simulink model "AirplaneSimModel_AutomaticTrajectory"  (R2018b)
settings: Solver=ode4  StartTime=0.0  StopTime=30  FixedStep=0.001  RelTol=1e-3
undefined symbols (not defined in the file): aileron_left, aileron_right, airplane, alt_ground, atmosphere, B_aileron_p_14ms, B_elevator_q_14ms, B_rudder_r_14ms, elevator, envir, g, htp_trim, inital_vel_vec, K_atti, K_lateral, K_vertical, rudder, throttle, traj, wind
libraries: actuators_lib x11, unit_conversions_lib x6, axes_transformation_lib x2, quatAttitudeController_lib x2, conventional_airplane_single_engine_lib x1, atmosphere_lib x1, sensors_lib x1, simulink x1, flightgear_visualization_lib x1
(part 1 of 2)
settings Model: Creator=Fgücker  LastModifiedBy=fabian

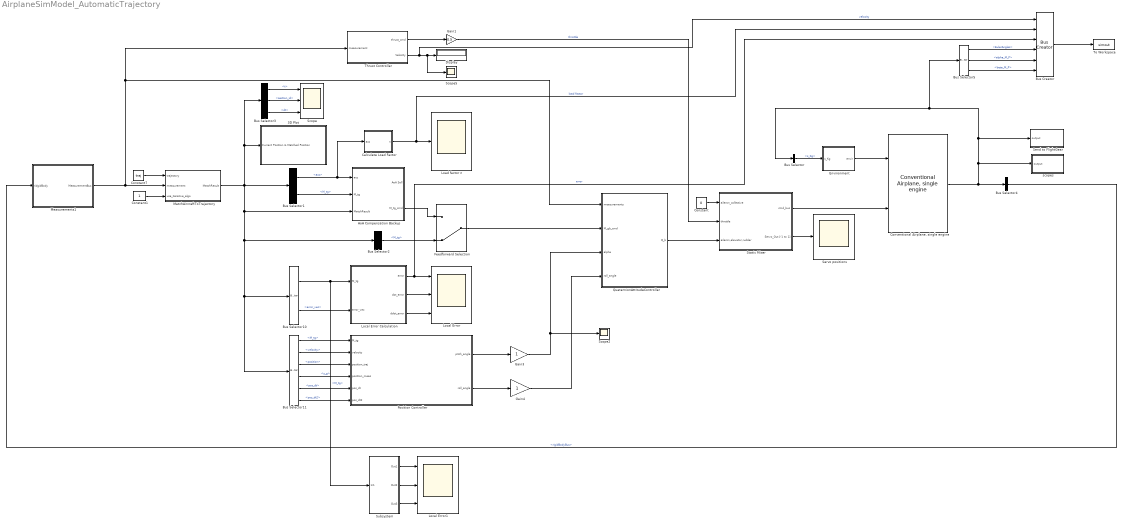
== system AirplaneSimModel_AutomaticTrajectory ==
  3D Plot : Subsystem
  AoA Compensation Backup : Subsystem
  Bus Creator : BusCreator  Inputs=6
  Bus Selector : BusSelector  OutputSignals=rigidBodyBus.s_Kg
  Bus Selector1 : BusSelector  OutputSignals=acc,M_tg
  Bus Selector10 : BusSelector  OutputSignals=M_tg,error_vec
  Bus Selector11 : BusSelector  OutputSignals=M_tg,velocity,position,s_g,pos_dt,pos_dt2
  Bus Selector2 : BusSelector  OutputSignals=M_tg
  Bus Selector3 : BusSelector  OutputSignals=t,section_id,dt
  Bus Selector4 : BusSelector  OutputSignals=rigidBodyBus
  Bus Selector5 : BusSelector  OutputSignals=rigidBodyBus.EulerAngles,aeroBus.aeroMainWing.aeroAxes.alpha_M_P,aeroBus.aeroMainWing.aeroAxes.beta_M_P
  Calculate Load Factor : Subsystem
  Constant : Constant  Value=0
  Constant1 : Constant
  Constant7 : Constant  Value=traj  OutDataTypeStr=Bus: trajectoryBus
  "Conventional Airplane, single engine" : conventional_airplane_single_engine_lib/Conventional Airplane, single engine  airplane=airplane
      settings: SourceProductName=LADAC
  Display : Display
  Environment : Subsystem
  Feedforward Selection : ManualSwitch  CurrentSetting=0
  Gain1 : Gain  Gain=0.5
  Gain3 : Gain
  Gain4 : Gain
  Load factor n : Scope
  Local Error : Scope  NumInputPorts=3
  Local Error Calculation : Subsystem
  Local Error1 : Scope  NumInputPorts=3
  MatchAircraftToTrajectory : Subsystem
  Measurements1 : Subsystem  mask{omega0=80, D=1}
      mask prompts: omega0 "Omega - Filter"; D "Damping D - Filter"
  Position Controller : Subsystem
  QuaternionAttitudeController : Subsystem
  Scope : Scope  NumInputPorts=3
  Scope2 : Scope
  Scope5 : Scope
  Send to FlightGear : Subsystem
  Servo positions : Scope
  Static Mixer : Subsystem
  Subsystem : Subsystem
  Thrust Controller : Subsystem
  To Workspace : ToWorkspace  VariableName=simout  SaveFormat=Timeseries  SampleTime=-1
  scopes : Subsystem
  wires:
  Bus Selector4/1 -> Measurements1/1(ridgidBody)  "<rigidBodyBus>"
  Measurements1/1(MeasurementBus) -> Thrust Controller/1(measurement), QuaternionAttitudeController/1(measurements), MatchAircraftToTrajectory/2(measurement)
  Thrust Controller/1(thrust_cmd) -> Gain1/1
  Thrust Controller/2(Velocity) -> Bus Creator/1, Scope5/1, Display/1  "velocity"
  AoA Compensation Backup/2(M_tg_cmd) -> Feedforward Selection/1
  "Conventional Airplane, single engine"/1 -> Bus Selector4/1, Bus Selector5/1, Bus Selector/1, Send to FlightGear/1(output), scopes/1(output)
  Environment/1(envir) -> "Conventional Airplane, single engine"/1
  Bus Selector/1 -> Environment/1(s_Kg)  "<s_Kg>"
  Feedforward Selection/1 -> QuaternionAttitudeController/2(M_gb_cmd)
  Bus Selector11/2 -> Position Controller/2(velocity)  "<velocity>"
  Bus Selector11/3 -> Position Controller/3(position_traj)  "<position>"
  Local Error Calculation/3(ddot_error) -> Local Error/3
  Local Error Calculation/2(dot_error) -> Local Error/2
  Local Error Calculation/1(error) -> Bus Creator/3, Local Error/1  "error"
  Bus Selector10/2 -> Local Error Calculation/2(error_vec)  "<error_vec>"
  Gain1/1 -> Static Mixer/2(throttle)  "throttle"
  QuaternionAttitudeController/1(Q_b) -> Static Mixer/3(aileron,elevator,rudder)
  Static Mixer/1(cmd_bus) -> "Conventional Airplane, single engine"/2
  Static Mixer/2(Servo_Out [-1 to 1]) -> Servo positions/1
  Constant7/1 -> MatchAircraftToTrajectory/1(trajectory)
  Bus Selector11/1 -> Position Controller/1(M_tg)  "<M_tg>"
  Bus Selector10/1 -> Subsystem/1(In1), Local Error Calculation/1(M_tg)  "<M_tg>"
  Bus Selector11/4 -> Position Controller/4(position_meas)  "<s_g>"
  Calculate Load Factor/1(n) -> Bus Creator/2, Load factor n/1  "load factor"
  Bus Selector1/1 -> AoA Compensation Backup/1(acc), Calculate Load Factor/1(acc)  "<acc>"
  Bus Selector1/2 -> AoA Compensation Backup/2(M_tg)  "<M_tg>"
  Bus Selector2/1 -> Feedforward Selection/2  "<M_tg>"
  Constant/1 -> Static Mixer/1(aileron_collective)
  Bus Selector3/1 -> Scope/1  "<t>"
  Bus Selector3/2 -> Scope/2  "<section_id>"
  Subsystem/1(Out1) -> Local Error1/1
  Subsystem/2(Out2) -> Local Error1/2
  Subsystem/3(Out3) -> Local Error1/3
  Gain3/1 -> Scope2/1, QuaternionAttitudeController/3(alpha)
  Gain4/1 -> QuaternionAttitudeController/4(roll_angle)
  Bus Creator/1 -> To Workspace/1
  Bus Selector5/1 -> Bus Creator/4  "<EulerAngles>"
  Bus Selector5/2 -> Bus Creator/5  "<alpha_M_P>"
  Bus Selector5/3 -> Bus Creator/6  "<beta_M_P>"
  Constant1/1 -> MatchAircraftToTrajectory/3(use_iterative_algo)
  Bus Selector11/5 -> Position Controller/5(pos_dt)  "<pos_dt>"
  Bus Selector11/6 -> Position Controller/6(pos_dt2)  "<pos_dt2>"
  MatchAircraftToTrajectory/1(MatchResult) -> Bus Selector11/1, Bus Selector10/1, Bus Selector2/1, AoA Compensation Backup/3(MatchResult), Bus Selector1/1, Bus Selector3/1, 3D Plot/1(Current Position & Matched Position)
  Position Controller/1(pitch_angle) -> Gain3/1
  Position Controller/2(roll_angle) -> Gain4/1
  Bus Selector3/3 -> Scope/3  "<dt>"

== system AirplaneSimModel_AutomaticTrajectory/3D Plot ==
  Current Position & Matched Position : Inport
  3D Graph : S-Function  LoadFcn=if exist('sfun3d','file'), sfun3d([],[],[],'LoadBlock'); end  FunctionName=sfun3d  Parameters=ax,T,np,cp,gd,ls,mk,mx,hd,tb  SFunctionDeploymentMode=off  EnableBusSupport=off  mask(3D Graph){np=2, ax=[-8 8 -8 8 -8 8]*20, mx=1e4, T=0.040, cp=[-1 -1 1]*35, gd=on, hd=off, tb=off, ls=-, mk=none}
      mask prompts: np "Number of moving points (lines)"; ax "Range: [xmin xmax  ymin ymax zmin zmax]"; mx "Max number of points in each line"; T "Sampling Time"; cp "Camera position (use [0 0 1] for 2D XY view)"; gd "Grid (on|off)"; hd "HeadMarkers (on|off)"; tb "Toolbar (on|off)"; ls "LineStyle"; mk "LineMarker"
      mask help:
      | This block plots the position of several points in the XYZ space. The input contains the coordinates of all the points (x1,y1,z1,x2,y2,z2,...).
      | The number of moving points (lines), the XYZ ranges, sampling time, camera position, and grid (among other things) can be set as mask parameters.
      settings: CopyFcn=if exist('sfun3d','file'), sfun3d([],[],[],'CopyBlock'); end  DeleteFcn=if exist('sfun3d','file'), sfun3d([],[],[],'DeleteBlock'); end  NameChangeFcn=if exist('sfun3d','file'), sfun3d([],[],[],'NameChange'); end
      mask Help:
      | This block plots the position of several points in the XYZ space. The input contains the coordinates of all the points (x1,y1,z1,x2,y2,z2,...).
      | The number of moving points (lines), the XYZ ranges, sampling time, camera position, and grid (among other things) can be set as mask parameters.
      mask TypeOptions ls: - | -- | : | -. | none
      mask TypeOptions mk: none | . | + | o | * | x | square | diamond | v | ^ | > | < | pentagram | hexagram
      mask Display: plot([.05 .95 .95 .05 .05],[.45 .45 .95 .95 .45], 0.5+cos(0:0.1:2*pi)*0.3,0.7+sin(0:0.1:2*pi)*0.2)
  Bus Selector5 : BusSelector  OutputSignals=s_g,position
  Gain19 : Gain  Gain=[1 1 -1]'
  Gain2 : Gain  Gain=[1 1 -1]'
  Mux : Mux  Inputs=2
  wires:
  Bus Selector5/2 -> Gain19/1  "<position>"
  Gain19/1 -> Mux/2
  Current Position & Matched Position/1 -> Bus Selector5/1
  Bus Selector5/1 -> Gain2/1  "<s_g>"
  Mux/1 -> 3D Graph/1
  Gain2/1 -> Mux/1

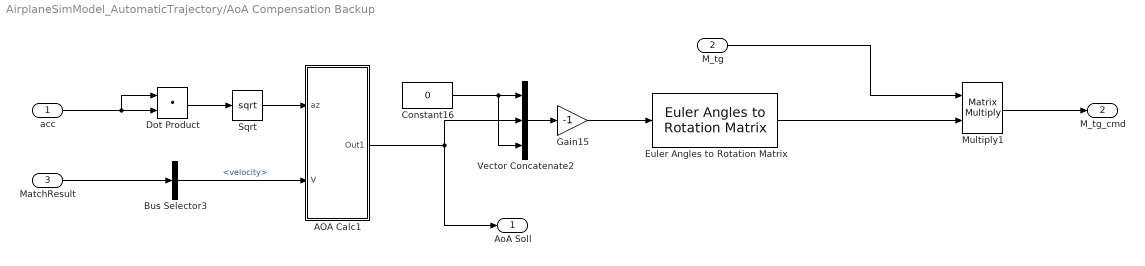
== system AirplaneSimModel_AutomaticTrajectory/AoA Compensation Backup ==
  acc : Inport
  M_tg : Inport  Port=2
  MatchResult : Inport  Port=3
  AOA Calc1 : Subsystem
  Bus Selector3 : BusSelector  OutputSignals=velocity
  Constant16 : Constant  Value=0
  Dot Product : DotProduct  InputSameDT=on  OutDataTypeStr=Inherit: Inherit via internal rule
  Euler Angles to Rotation Matrix : axes_transformation_lib/Euler Angles to Rotation Matrix  SystemSampleTime=-1
      settings: SourceProductName=LADAC
  Gain15 : Gain  Gain=-1
  Multiply1 : Product  Multiplication=Matrix(*)
  Sqrt : Sqrt  SaturateOnIntegerOverflow=on
  Vector Concatenate2 : Concatenate  NumInputs=3
  AoA Soll : Outport
  M_tg_cmd : Outport  Port=2
  wires:
  Bus Selector3/1 -> AOA Calc1/2(V)  "<velocity>"
  acc/1 -> Dot Product/2, Dot Product/1
  AOA Calc1/1(Out1) -> AoA Soll/1, Vector Concatenate2/2
  Sqrt/1 -> AOA Calc1/1(az)
  Constant16/1 -> Vector Concatenate2/3, Vector Concatenate2/1
  Euler Angles to Rotation Matrix/1 -> Multiply1/2
  Vector Concatenate2/1 -> Gain15/1
  Gain15/1 -> Euler Angles to Rotation Matrix/1
  MatchResult/1 -> Bus Selector3/1
  M_tg/1 -> Multiply1/1
  Multiply1/1 -> M_tg_cmd/1
  Dot Product/1 -> Sqrt/1

== system AirplaneSimModel_AutomaticTrajectory/Calculate Load Factor ==
  acc : Inport
  Dot Product : DotProduct  InputSameDT=on  OutDataTypeStr=Inherit: Inherit via internal rule
  Gain7 : Gain  Gain=1/g
  Sqrt : Sqrt  SaturateOnIntegerOverflow=on
  n : Outport
  wires:
  Dot Product/1 -> Sqrt/1
  Sqrt/1 -> Gain7/1
  acc/1 -> Dot Product/1, Dot Product/2
  Gain7/1 -> n/1

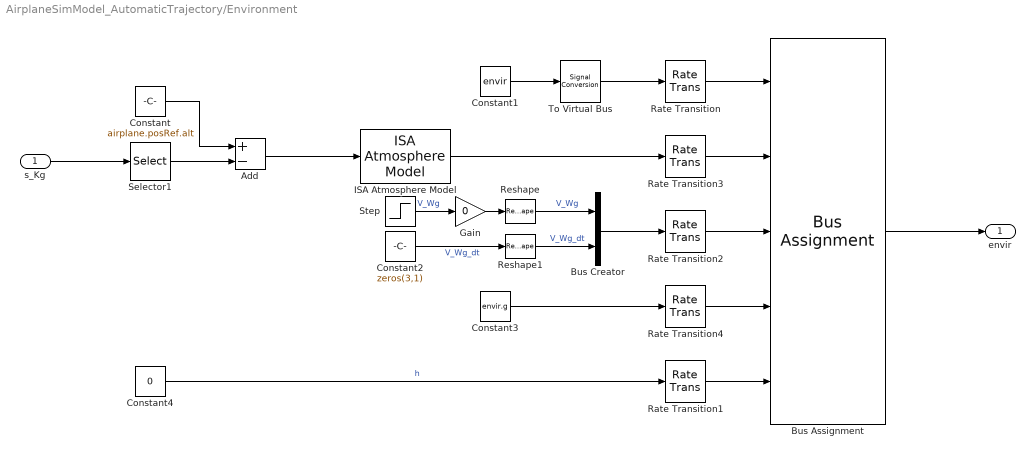
== system AirplaneSimModel_AutomaticTrajectory/Environment ==
  s_Kg : Inport
  Add : Sum  Inputs=+-
  Bus Assignment : BusAssignment  AssignedSignals=atmosphere,wind,g,alt_ground
  Bus Creator : BusCreator  Inputs=2
  Constant : Constant  Value=airplane.posRef.alt
  Constant1 : Constant  Value=envir  OutDataTypeStr=Bus: envirBus
  Constant2 : Constant  Value=zeros(3,1)
  Constant3 : Constant  Value=envir.g
  Constant4 : Constant  Value=0
  Gain : Gain  Gain=0
  ISA Atmosphere Model : atmosphere_lib/ISA Atmosphere Model  SystemSampleTime=-1
      settings: SourceProductName=LADAC
  Rate Transition{,1..4} (5 alike) : RateTransition
  Reshape : Reshape  OutputDimensionality=Column vector (2-D)
  Reshape1 : Reshape  OutputDimensionality=Column vector (2-D)
  Selector1 : Selector  InputPortWidth=3  IndexOptions=Index vector (dialog)  Indices=3  OutputSizes=1
  Step : Step  Time=3  After=[0;10;0]  SampleTime=0
  To Virtual Bus : SignalConversion  ConversionOutput=Virtual bus  OverrideOpt=off
  envir : Outport
  wires:
  Constant4/1 -> Rate Transition1/1  "h"
  Rate Transition2/1 -> Bus Assignment/3
  Rate Transition3/1 -> Bus Assignment/2
  Bus Assignment/1 -> envir/1
  Rate Transition/1 -> Bus Assignment/1
  ISA Atmosphere Model/1 -> Rate Transition3/1
  Step/1 -> Gain/1  "V_Wg"
  Rate Transition1/1 -> Bus Assignment/5
  Constant1/1 -> To Virtual Bus/1
  s_Kg/1 -> Selector1/1
  Bus Creator/1 -> Rate Transition2/1
  Constant2/1 -> Reshape1/1  "V_Wg_dt"
  Rate Transition4/1 -> Bus Assignment/4
  Constant3/1 -> Rate Transition4/1
  Gain/1 -> Reshape/1
  Constant/1 -> Add/1
  Add/1 -> ISA Atmosphere Model/1
  Selector1/1 -> Add/2
  To Virtual Bus/1 -> Rate Transition/1
  Reshape/1 -> Bus Creator/1  "V_Wg"
  Reshape1/1 -> Bus Creator/2  "V_Wg_dt"

== system AirplaneSimModel_AutomaticTrajectory/Local Error Calculation ==
  M_tg : Inport
  error_vec : Inport  Port=2
  Derivative1 : Derivative
  Derivative2 : Derivative
  Multiply2 : Product  Multiplication=Matrix(*)
  Transpose : Math  Operator=transpose  SaturateOnIntegerOverflow=on
  error : Outport
  dot_error : Outport  Port=2
  ddot_error : Outport  Port=3
  wires:
  error_vec/1 -> Multiply2/2
  Transpose/1 -> Multiply2/1
  M_tg/1 -> Transpose/1
  Derivative1/1 -> dot_error/1, Derivative2/1
  Derivative2/1 -> ddot_error/1
  Multiply2/1 -> Derivative1/1, error/1

== system AirplaneSimModel_AutomaticTrajectory/MatchAircraftToTrajectory ==
  trajectory : Inport
  measurement : Inport  Port=2
  use_iterative_algo : Inport  Port=3
  Bus Creator : BusCreator  Inputs=13
  Bus Selector1 : BusSelector  OutputSignals=EKF.s_g,EKF.velocity
  Bus Selector3 : BusSelector  OutputSignals=EKF.s_g,EKF.velocity
  Constant : Constant  Value=[0; 0; -g]  VectorParams1D=off
  Derivative : Derivative
  MATLAB Function6 : MATLAB Function  TreatAsAtomicUnit=on
  MatchResult : Outport
  wires:
  Bus Selector3/1 -> MATLAB Function6/2(pos_ac)  "<s_g>"
  trajectory/1 -> MATLAB Function6/1(traj)  "trajectory"
  measurement/1 -> Bus Selector1/1, Bus Selector3/1
  Bus Creator/1 -> MatchResult/1
  Bus Selector3/2 -> MATLAB Function6/3(vel), Derivative/1  "<velocity>"
  MATLAB Function6/1(pos) -> Bus Creator/1  "position"
  MATLAB Function6/2(error) -> Bus Creator/2  "error_norm"
  MATLAB Function6/3(error_vec) -> Bus Creator/3  "error_vec"
  MATLAB Function6/4(section_idx) -> Bus Creator/4  "section_id"
  MATLAB Function6/5(t) -> Bus Creator/5  "t"
  Constant/1 -> MATLAB Function6/5(acc_vec)
  MATLAB Function6/6(acc) -> Bus Creator/6  "acc"
  MATLAB Function6/7(M_tg) -> Bus Creator/7  "M_tg"
  use_iterative_algo/1 -> MATLAB Function6/6(use_iterative_algo)
  MATLAB Function6/8(dt) -> Bus Creator/8
  MATLAB Function6/9(pos_dt) -> Bus Creator/9
  MATLAB Function6/10(pos_dt2) -> Bus Creator/10
  Derivative/1 -> MATLAB Function6/4(vel_dt)
  Bus Selector1/1 -> Bus Creator/12  "<s_g>"
  Bus Selector1/2 -> Bus Creator/13  "<velocity>"

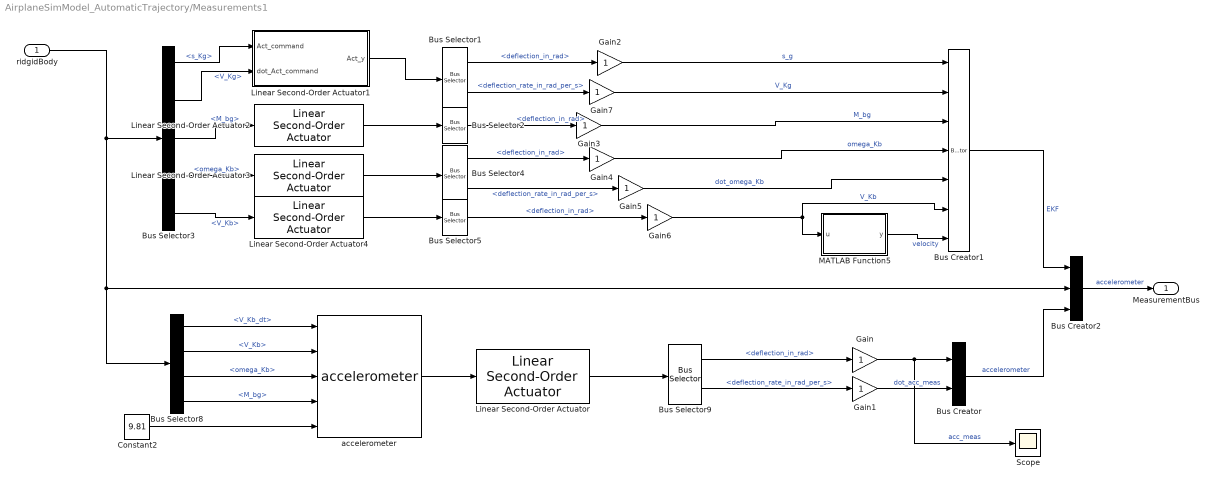
== system AirplaneSimModel_AutomaticTrajectory/Measurements1 ==
  ridgidBody : Inport
  Bus Creator : BusCreator  Inputs=2
  Bus Creator1 : BusCreator  Inputs=7
  Bus Creator2 : BusCreator  Inputs=3
  Bus Selector1 : BusSelector  OutputSignals=deflection_in_rad,deflection_rate_in_rad_per_s
  Bus Selector2 : BusSelector  OutputSignals=deflection_in_rad
  Bus Selector3 : BusSelector  OutputSignals=s_Kg,V_Kg,M_bg,omega_Kb,V_Kb
  Bus Selector4 : BusSelector  OutputSignals=deflection_in_rad,deflection_rate_in_rad_per_s
  Bus Selector5 : BusSelector  OutputSignals=deflection_in_rad
  Bus Selector8 : BusSelector  OutputSignals=V_Kb_dt,V_Kb,omega_Kb,M_bg
  Bus Selector9 : BusSelector  OutputSignals=deflection_in_rad,deflection_rate_in_rad_per_s
  Constant2 : Constant  Value=9.81
  Gain{,1..7} (8 alike) : Gain
  Linear Second-Order Actuator : actuators_lib/Linear Second-Order Actuator  omega=omega0  d=D  A_0=[0 0 -g]  dot_A_0=0  start_steady_state=off
      settings: SourceProductName=LADAC
  Linear Second-Order Actuator1 : Subsystem  mask{omega=omega0, d=D, A_0=0, dot_A_0=0}
      mask prompts: omega "Natural frequency"; d "Damping ratio"; A_0 "Initial position"; dot_A_0 "Initial velocity"
  Linear Second-Order Actuator2 : actuators_lib/Linear Second-Order Actuator  omega=omega0  d=D  A_0=0  dot_A_0=0  start_steady_state=on
      settings: SourceProductName=LADAC
  Linear Second-Order Actuator3 : actuators_lib/Linear Second-Order Actuator  omega=omega0  d=D  A_0=0  dot_A_0=0  start_steady_state=on
      settings: SourceProductName=LADAC
  Linear Second-Order Actuator4 : actuators_lib/Linear Second-Order Actuator  omega=omega0  d=D  A_0=0  dot_A_0=0  start_steady_state=on
      settings: SourceProductName=LADAC
  MATLAB Function5 : MATLAB Function  TreatAsAtomicUnit=on
  Scope : Scope
  accelerometer : sensors_lib/accelerometer  SystemSampleTime=-1
  MeasurementBus : Outport
  wires:
  Bus Selector9/2 -> Gain1/1  "<deflection_rate_in_rad_per_s>"
  Bus Selector8/1 -> accelerometer/1  "<V_Kb_dt>"
  Linear Second-Order Actuator/1 -> Bus Selector9/1
  Bus Selector8/2 -> accelerometer/2  "<V_Kb>"
  Bus Selector8/3 -> accelerometer/3  "<omega_Kb>"
  Constant2/1 -> accelerometer/5
  Bus Selector8/4 -> accelerometer/4  "<M_bg>"
  accelerometer/1 -> Linear Second-Order Actuator/1
  Bus Selector9/1 -> Gain/1  "<deflection_in_rad>"
  Gain/1 -> Scope/1, Bus Creator/1  "acc_meas"
  Gain1/1 -> Bus Creator/2  "dot_acc_meas"
  ridgidBody/1 -> Bus Creator2/2, Bus Selector8/1, Bus Selector3/1
  Linear Second-Order Actuator1/1(Act_y) -> Bus Selector1/1
  Bus Selector3/1 -> Linear Second-Order Actuator1/1(Act_command)  "<s_Kg>"
  Bus Creator1/1 -> Bus Creator2/1  "EKF"
  Bus Creator2/1 -> MeasurementBus/1  "accelerometer"
  Bus Selector1/1 -> Gain2/1  "<deflection_in_rad>"
  Bus Selector3/3 -> Linear Second-Order Actuator2/1  "<M_bg>"
  Bus Selector3/4 -> Linear Second-Order Actuator3/1  "<omega_Kb>"
  Linear Second-Order Actuator2/1 -> Bus Selector2/1
  Linear Second-Order Actuator3/1 -> Bus Selector4/1
  Bus Selector4/2 -> Gain5/1  "<deflection_rate_in_rad_per_s>"
  Bus Selector4/1 -> Gain4/1  "<deflection_in_rad>"
  Bus Selector2/1 -> Gain3/1  "<deflection_in_rad>"
  Gain3/1 -> Bus Creator1/3  "M_bg"
  Gain4/1 -> Bus Creator1/4  "omega_Kb"
  Gain5/1 -> Bus Creator1/5  "dot_omega_Kb"
  Bus Selector3/5 -> Linear Second-Order Actuator4/1  "<V_Kb>"
  Linear Second-Order Actuator4/1 -> Bus Selector5/1
  Bus Selector5/1 -> Gain6/1  "<deflection_in_rad>"
  Gain6/1 -> MATLAB Function5/1(u), Bus Creator1/6  "V_Kb"
  Gain7/1 -> Bus Creator1/2  "V_Kg"
  MATLAB Function5/1(y) -> Bus Creator1/7  "velocity"
  Bus Creator/1 -> Bus Creator2/3  "accelerometer"
  Gain2/1 -> Bus Creator1/1  "s_g"
  Bus Selector1/2 -> Gain7/1  "<deflection_rate_in_rad_per_s>"
  Bus Selector3/2 -> Linear Second-Order Actuator1/2(dot_Act_command)  "<V_Kg>"

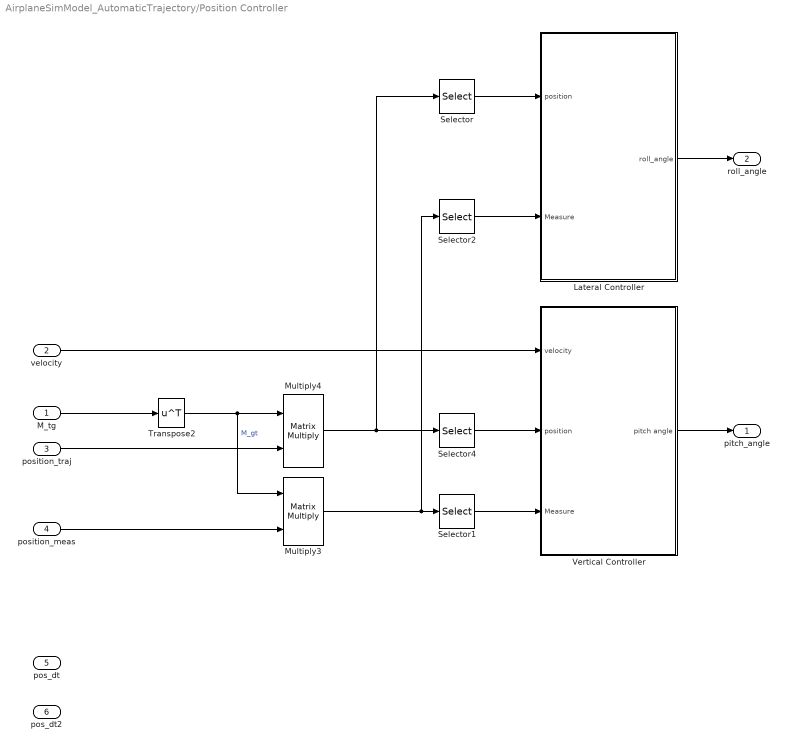
== system AirplaneSimModel_AutomaticTrajectory/Position Controller ==
  M_tg : Inport
  velocity : Inport  Port=2
  position_traj : Inport  Port=3
  position_meas : Inport  Port=4
  pos_dt : Inport  Port=5
  pos_dt2 : Inport  Port=6
  Lateral Controller : Subsystem
  Multiply3 : Product  Multiplication=Matrix(*)
  Multiply4 : Product  Multiplication=Matrix(*)
  Selector : Selector  InputPortWidth=3  IndexOptions=Index vector (dialog)  Indices=2  OutputSizes=1
  Selector1 : Selector  InputPortWidth=3  IndexOptions=Index vector (dialog)  Indices=3  OutputSizes=1
  Selector2 : Selector  InputPortWidth=3  IndexOptions=Index vector (dialog)  Indices=2  OutputSizes=1
  Selector4 : Selector  InputPortWidth=3  IndexOptions=Index vector (dialog)  Indices=3  OutputSizes=1
  Transpose2 : Math  Operator=transpose  SaturateOnIntegerOverflow=on
  Vertical Controller : Subsystem
  pitch_angle : Outport
  roll_angle : Outport  Port=2
  wires:
  position_meas/1 -> Multiply3/2
  Multiply4/1 -> Selector/1, Selector4/1
  Vertical Controller/1(pitch angle) -> pitch_angle/1
  Transpose2/1 -> Multiply4/1, Multiply3/1  "M_gt"
  M_tg/1 -> Transpose2/1
  velocity/1 -> Vertical Controller/1(velocity)
  Multiply3/1 -> Selector2/1, Selector1/1
  position_traj/1 -> Multiply4/2
  Selector/1 -> Lateral Controller/1(position)
  Selector2/1 -> Lateral Controller/2(Measure)
  Lateral Controller/1(roll_angle) -> roll_angle/1
  Selector4/1 -> Vertical Controller/2(position)
  Selector1/1 -> Vertical Controller/3(Measure)

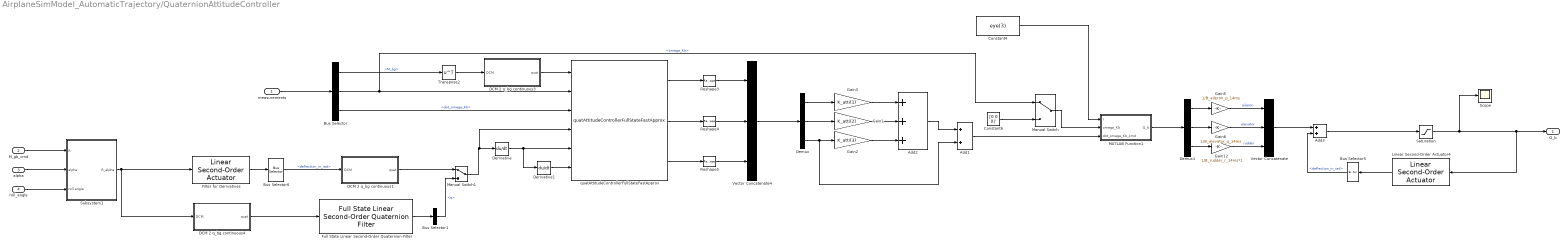
== system AirplaneSimModel_AutomaticTrajectory/QuaternionAttitudeController ==
  measurements : Inport
  M_gb_cmd : Inport  Port=2
  alpha : Inport  Port=3
  roll_angle : Inport  Port=4
  Add1 : Sum
  Add2 : Sum  Inputs=+++
  Add3 : Sum
  Bus Selector : BusSelector  OutputSignals=EKF.M_bg,EKF.omega_Kb,EKF.dot_omega_Kb
  Bus Selector1 : BusSelector  OutputSignals=q
  Bus Selector5 : BusSelector  OutputSignals=deflection_in_rad
  Bus Selector6 : BusSelector  OutputSignals=deflection_in_rad
  Constant4 : Constant  Value=eye(3)  VectorParams1D=off
  Constant6 : Constant  Value=[0 0 0]'  VectorParams1D=off
  DCM 2 q_bg continuous1 : Subsystem
      mask DialogControl DescGroupVar Prompt: Get quaternions from DCM without discontinuities
      mask DialogControl DescTextVar Prompt: Look inside the block (and function) for more information.
  DCM 2 q_bg continuous3 : Subsystem
      mask DialogControl DescGroupVar Prompt: Get quaternions from DCM without discontinuities
      mask DialogControl DescTextVar Prompt: Look inside the block (and function) for more information.
  DCM 2 q_bg continuous4 : Subsystem
      mask DialogControl DescGroupVar Prompt: Get quaternions from DCM without discontinuities
      mask DialogControl DescTextVar Prompt: Look inside the block (and function) for more information.
  Demux : Demux  Outputs=3
  Demux1 : Demux  Outputs=3
  Derivative : Derivative
  Derivative1 : Derivative
  Filter for Derivatives : actuators_lib/Linear Second-Order Actuator  omega=200  d=1  A_0=0  dot_A_0=0  start_steady_state=off
      settings: SourceProductName=LADAC
  Full State Linear Second-Order Quaternion Filter : quatAttitudeController_lib/Full State Linear Second-Order Quaternion Filter  omega_0=200  D=1  q_0=[1; 0; 0; 0]  omega_Kb_0=[0; 0; 0]
      settings: SourceProductName=LADAC
  Gain1 : Gain  Gain=K_atti(2)
  Gain12 : Gain  Gain=1/B_rudder_r_14ms*1
  Gain2 : Gain  Gain=K_atti(3)
  Gain3 : Gain  Gain=K_atti(1)
  Gain5 : Gain  Gain=1/B_aileron_p_14ms
  Gain6 : Gain  Gain=1/B_elevator_q_14ms
  Linear Second-Order Actuator4 : actuators_lib/Linear Second-Order Actuator  omega=40  d=1  A_0=[0 0 0]'  dot_A_0=0  start_steady_state=off
      settings: SourceProductName=LADAC
  MATLAB Function1 : MATLAB Function  TreatAsAtomicUnit=on
  Manual Switch : ManualSwitch
  Manual Switch1 : ManualSwitch
  Reshape3 : Reshape  OutputDimensionality=Column vector (2-D)
  Reshape4 : Reshape  OutputDimensionality=Column vector (2-D)
  Reshape5 : Reshape  OutputDimensionality=Column vector (2-D)
  Saturation : Saturate  UpperLimit=1  LowerLimit=-1
  Scope : Scope
  Subsystem1 : Subsystem
  Transpose2 : Math  Operator=transpose  SaturateOnIntegerOverflow=on
  Vector Concatenate : Concatenate  NumInputs=3
  Vector Concatenate4 : Concatenate  NumInputs=3
  quatAttitudeControllerFullStateFastApprox : quatAttitudeController_lib/quatAttitudeControllerFullStateFastApprox  SystemSampleTime=-1
      settings: SourceProductName=LADAC
  Q_b : Outport
  wires:
  Bus Selector/3 -> quatAttitudeControllerFullStateFastApprox/3  "<dot_omega_Kb>"
  Derivative1/1 -> quatAttitudeControllerFullStateFastApprox/6
  Filter for Derivatives/1 -> Bus Selector6/1
  Vector Concatenate4/1 -> Demux/1
  Bus Selector/2 -> Manual Switch/1, quatAttitudeControllerFullStateFastApprox/2  "<omega_Kb>"
  Manual Switch/1 -> MATLAB Function1/2(omega_Kb)
  Gain3/1 -> Add2/1
  Derivative/1 -> Derivative1/1, quatAttitudeControllerFullStateFastApprox/5
  Gain1/1 -> Add2/2
  Demux/3 -> Add1/2, Gain2/1
  Add2/1 -> Add1/1
  Constant6/1 -> Manual Switch/2
  Constant4/1 -> MATLAB Function1/1(I)
  measurements/1 -> Bus Selector/1
  MATLAB Function1/1(Q_b) -> Demux1/1
  Bus Selector/1 -> Transpose2/1  "<M_bg>"
  DCM 2 q_bg continuous3/1(quat) -> quatAttitudeControllerFullStateFastApprox/1
  quatAttitudeControllerFullStateFastApprox/1 -> Reshape3/1
  Reshape3/1 -> Vector Concatenate4/1
  Reshape4/1 -> Vector Concatenate4/2
  Reshape5/1 -> Vector Concatenate4/3
  quatAttitudeControllerFullStateFastApprox/3 -> Reshape5/1
  M_gb_cmd/1 -> Subsystem1/1(R)
  alpha/1 -> Subsystem1/2(alpha)
  Bus Selector6/1 -> DCM 2 q_bg continuous1/1(DCM)  "<deflection_in_rad>"
  quatAttitudeControllerFullStateFastApprox/2 -> Reshape4/1
  roll_angle/1 -> Subsystem1/3(roll angle)
  Demux/1 -> Gain3/1
  Gain2/1 -> Add2/3
  Demux/2 -> Gain1/1
  Gain5/1 -> Vector Concatenate/1  "aileron"
  Gain6/1 -> Vector Concatenate/2  "elevator"
  Gain12/1 -> Vector Concatenate/3  "rudder"
  Demux1/1 -> Gain5/1
  Demux1/2 -> Gain6/1
  Demux1/3 -> Gain12/1
  Saturation/1 -> Scope/1, Q_b/1, Linear Second-Order Actuator4/1
  Bus Selector5/1 -> Add3/2  "<deflection_in_rad>"
  Vector Concatenate/1 -> Add3/1
  Linear Second-Order Actuator4/1 -> Bus Selector5/1
  Add3/1 -> Saturation/1
  Add1/1 -> MATLAB Function1/3(dot_omega_Kb_cmd)
  Full State Linear Second-Order Quaternion Filter/1 -> Bus Selector1/1
  DCM 2 q_bg continuous1/1(quat) -> Manual Switch1/1
  Bus Selector1/1 -> Manual Switch1/2  "<q>"
  Manual Switch1/1 -> quatAttitudeControllerFullStateFastApprox/4, Derivative/1
  Subsystem1/1(R_alpha) -> Filter for Derivatives/1, DCM 2 q_bg continuous4/1(DCM)
  DCM 2 q_bg continuous4/1(quat) -> Full State Linear Second-Order Quaternion Filter/1
  Transpose2/1 -> DCM 2 q_bg continuous3/1(DCM)

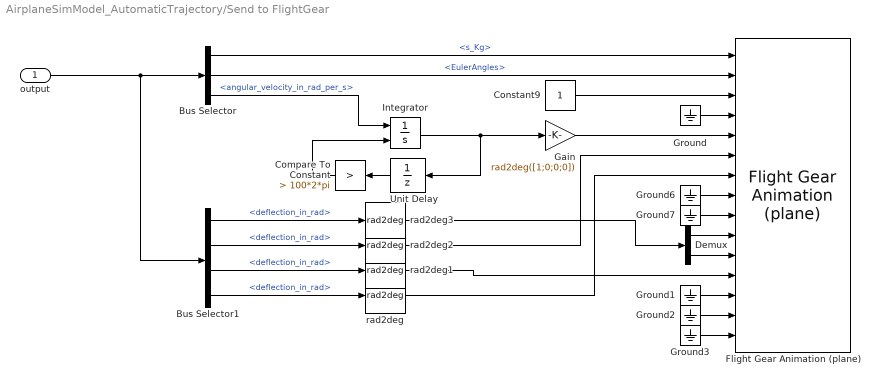
== system AirplaneSimModel_AutomaticTrajectory/Send to FlightGear ==
  output : Inport
  Bus Selector : BusSelector  OutputSignals=rigidBodyBus.s_Kg,rigidBodyBus.EulerAngles,actuatorBus.motorBus.angular_velocity_in_rad_per_s
  Bus Selector1 : BusSelector  OutputSignals=actuatorBus.aileronsBus.deflection_in_rad,actuatorBus.elevatorBus.deflection_in_rad,actuatorBus.rudderBus.deflection_in_rad,actuatorBus.htpTrimBus.deflection_in_rad
  Compare To Constant : simulink/Logic and Bit Operations/Compare To Constant  relop=>  const=100*2*pi  OutDataTypeStr=boolean
  Constant9 : Constant
  Demux : Demux  Outputs=2
  Flight Gear Animation (plane) : flightgear_visualization_lib/Flight Gear Animation (plane)  inital_lat=airplane.posRef.lat  inital_long=airplane.posRef.lon  inital_height=airplane.posRef.alt  remoteURL='127.0.0.1'  remotePort=5502
      settings: SourceProductName=LADAC
  Gain : Gain  Gain=rad2deg([1;0;0;0])
  Ground{,1..3,6..7} (6 alike) : Ground
  Integrator : Integrator  ExternalReset=rising
  Unit Delay : UnitDelay  SampleTime=-1
  rad2deg{,1..3} (4 alike) : unit_conversions_lib/rad2deg
      settings: SourceProductName=LADAC
  wires:
  Compare To Constant/1 -> Integrator/2
  Integrator/1 -> Unit Delay/1, Gain/1
  Bus Selector/1 -> Flight Gear Animation (plane)/1  "<s_Kg>"
  Bus Selector/2 -> Flight Gear Animation (plane)/2  "<EulerAngles>"
  Gain/1 -> Flight Gear Animation (plane)/5
  Constant9/1 -> Flight Gear Animation (plane)/3
  Unit Delay/1 -> Compare To Constant/1
  Ground/1 -> Flight Gear Animation (plane)/4
  Ground1/1 -> Flight Gear Animation (plane)/13
  Ground2/1 -> Flight Gear Animation (plane)/14
  Ground3/1 -> Flight Gear Animation (plane)/15
  output/1 -> Bus Selector1/1, Bus Selector/1
  Bus Selector/3 -> Integrator/1  "<angular_velocity_in_rad_per_s>"
  Bus Selector1/2 -> rad2deg2/1  "<deflection_in_rad>"
  Bus Selector1/4 -> rad2deg/1  "<deflection_in_rad>"
  Ground6/1 -> Flight Gear Animation (plane)/8
  Ground7/1 -> Flight Gear Animation (plane)/9
  Bus Selector1/3 -> rad2deg1/1  "<deflection_in_rad>"
  Bus Selector1/1 -> rad2deg3/1  "<deflection_in_rad>"
  Demux/1 -> Flight Gear Animation (plane)/10
  Demux/2 -> Flight Gear Animation (plane)/11
  rad2deg/1 -> Flight Gear Animation (plane)/7
  rad2deg1/1 -> Flight Gear Animation (plane)/12
  rad2deg2/1 -> Flight Gear Animation (plane)/6
  rad2deg3/1 -> Demux/1

== system AirplaneSimModel_AutomaticTrajectory/Static Mixer ==
  aileron_collective : Inport
  throttle : Inport  Port=2
  aileron,elevator,rudder : Inport  Port=3
  Assignment : Assignment  DiagnosticForDimensions=Warning  IndexOptions=Index vector (dialog)  Indices=[1,2,3,4,5]  OutputSizes=1
  Constant3 : Constant  Value=zeros(8,1)  VectorParams1D=off
  Demux : Demux  Outputs=3
  Vector Concatenate : Concatenate  NumInputs=5
  mixer : Subsystem
  cmd_bus : Outport
  Servo_Out [-1 to 1] : Outport  Port=2
  wires:
  Constant3/1 -> Assignment/1
  Demux/2 -> Vector Concatenate/2  "elevator"
  Demux/1 -> Vector Concatenate/1  "aileron"
  Assignment/1 -> mixer/1(cmd_01)
  Demux/3 -> Vector Concatenate/3  "rudder"
  mixer/1(Out1) -> cmd_bus/1
  aileron_collective/1 -> Vector Concatenate/5
  Vector Concatenate/1 -> Servo_Out [-1 to 1]/1, Assignment/2
  throttle/1 -> Vector Concatenate/4
  aileron,elevator,rudder/1 -> Demux/1

== system AirplaneSimModel_AutomaticTrajectory/Subsystem ==
  In1 : Inport
  Derivative1 : Derivative
  Derivative2 : Derivative
  Gain : Gain
  Out1 : Outport
  Out2 : Outport  Port=2
  Out3 : Outport  Port=3
  wires:
  In1/1 -> Gain/1
  Derivative2/1 -> Out3/1
  Gain/1 -> Out1/1, Derivative1/1
  Derivative1/1 -> Out2/1, Derivative2/1

== system AirplaneSimModel_AutomaticTrajectory/Thrust Controller ==
  measurement : Inport
  Add2 : Sum  Inputs=+-
  Bus Selector14 : BusSelector  OutputSignals=deflection_in_rad
  Bus Selector4 : BusSelector  OutputSignals=EKF.V_Kb
  Constant : Constant  Value=norm(inital_vel_vec)*1
  Linear Second-Order Actuator6 : actuators_lib/Linear Second-Order Actuator  omega=20  d=1.5  A_0=0  dot_A_0=0  start_steady_state=off
      settings: SourceProductName=LADAC
  Saturation3 : Saturate  UpperLimit=10  LowerLimit=0
  Selector : Selector  InputPortWidth=3  IndexOptions=Index vector (dialog)  Indices=1  OutputSizes=1
  thrust_cmd : Outport
  Velocity : Outport  Port=2
  wires:
  Linear Second-Order Actuator6/1 -> Bus Selector14/1
  Selector/1 -> Velocity/1, Add2/2
  Add2/1 -> Saturation3/1
  Constant/1 -> Add2/1
  Bus Selector4/1 -> Selector/1  "<V_Kb>"
  measurement/1 -> Bus Selector4/1
  Saturation3/1 -> Linear Second-Order Actuator6/1
  Bus Selector14/1 -> thrust_cmd/1  "<deflection_in_rad>"

== system AirplaneSimModel_AutomaticTrajectory/scopes ==
  output : Inport
  Bus Selector : BusSelector  OutputSignals=rigidBodyBus,aeroBus,actuatorBus
  actuator scopes : Subsystem
  aero scopes : Subsystem
  rigid body scopes : Subsystem
  wires:
  Bus Selector/1 -> rigid body scopes/1(rigidBodyBus)  "<rigidBodyBus>"
  Bus Selector/2 -> aero scopes/1(aeroBus)  "<aeroBus>"
  output/1 -> Bus Selector/1
  Bus Selector/3 -> actuator scopes/1(actuatorBus)  "<actuatorBus>"

== system AirplaneSimModel_AutomaticTrajectory/AoA Compensation Backup/AOA Calc1 ==
  az : Inport
  V : Inport  Port=2
  Constant12 : Constant  Value=1.225
  Constant14 : Constant  Value=0.3358
  Constant15 : Constant  Value=5.75
  Constant5 : Constant
  MATLAB Function : MATLAB Function  TreatAsAtomicUnit=on
  Out1 : Outport
  wires:
  Constant5/1 -> MATLAB Function/5(m)
  MATLAB Function/1(alpha) -> Out1/1
  V/1 -> MATLAB Function/1(V)
  az/1 -> MATLAB Function/4(az)
  Constant12/1 -> MATLAB Function/6(rho)
  Constant14/1 -> MATLAB Function/3(S)
  Constant15/1 -> MATLAB Function/2(C_A)

== system AirplaneSimModel_AutomaticTrajectory/Measurements1/Linear Second-Order Actuator1 ==
  Act_command : Inport
  dot_Act_command : Inport  Port=2
  2*d/omega : Gain  Gain=2*d/omega
  A : Integrator  InitialConditionSource=external  InitialCondition=A_0  ContinuousStateAttributes='A'
  Bus Creator : BusCreator  Inputs=3
  Sum2 : Sum  Inputs=|+-
  Sum3 : Sum  Inputs=|++
  dot_A : Integrator  InitialConditionSource=external  InitialCondition=dot_A_0  ContinuousStateAttributes='dot_A'
  omega^2 : Gain  Gain=omega^2
  Act_y : Outport
  wires:
  Bus Creator/1 -> Act_y/1
  omega^2/1 -> dot_A/1, Bus Creator/1  "deflection_acceleration_in_rad_per_square_s"
  Sum3/1 -> Sum2/2
  A/1 -> Sum3/1, Bus Creator/3  "deflection_in_rad"
  Sum2/1 -> omega^2/1
  Act_command/1 -> A/2, Sum2/1
  dot_A/1 -> A/1, Bus Creator/2, 2*d/omega/1  "deflection_rate_in_rad_per_s"
  2*d/omega/1 -> Sum3/2
  dot_Act_command/1 -> dot_A/2

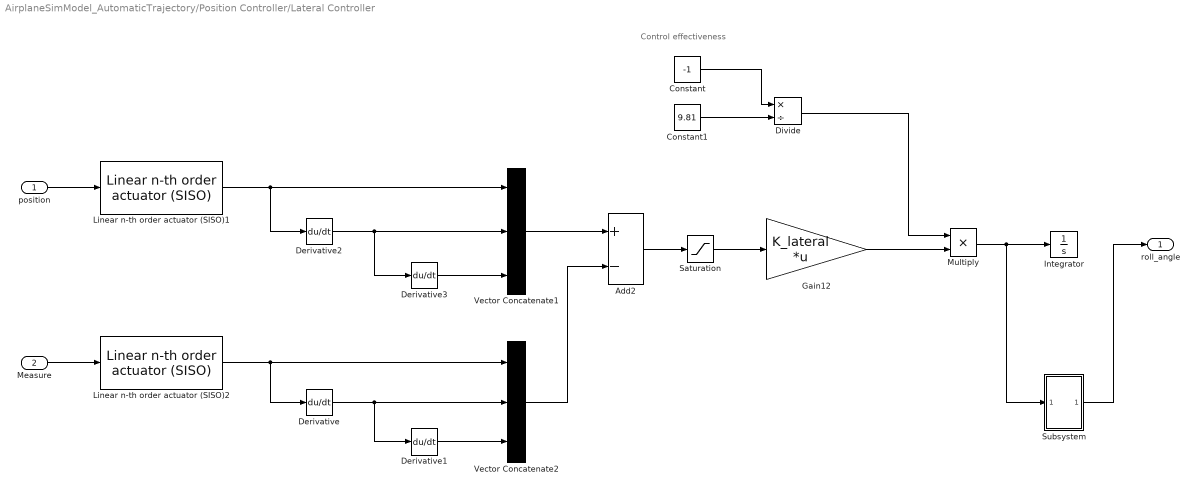
== system AirplaneSimModel_AutomaticTrajectory/Position Controller/Lateral Controller ==
  note: Control effectiveness
  position : Inport  PortDimensions=1
  Measure : Inport  Port=2
  Add2 : Sum  Inputs=+-
  Constant : Constant  Value=-1
  Constant1 : Constant  Value=9.81
  Derivative{,1..3} (4 alike) : Derivative
  Divide : Product  Inputs=*/
  Gain12 : Gain  Gain=K_lateral  Multiplication=Matrix(K*u)
  Integrator : Integrator
  Linear n-th order actuator (SISO)1 : actuators_lib/Linear n-th order actuator (SISO)  omega=80  order=2  output_order=1  use_inital_value=on
      settings: SourceProductName=LADAC
  Linear n-th order actuator (SISO)2 : actuators_lib/Linear n-th order actuator (SISO)  omega=80  order=2  output_order=1  use_inital_value=on
      settings: SourceProductName=LADAC
  Multiply : Product
  Saturation : Saturate  UpperLimit=[20 inf inf]  LowerLimit=-[20 inf inf]
  Subsystem : Subsystem
  Vector Concatenate1 : Concatenate  NumInputs=3
  Vector Concatenate2 : Concatenate  NumInputs=3
  roll_angle : Outport  PortDimensions=1
  wires:
  Derivative/1 -> Derivative1/1, Vector Concatenate2/2
  Constant/1 -> Divide/1
  Derivative1/1 -> Vector Concatenate2/3
  Divide/1 -> Multiply/1
  Gain12/1 -> Multiply/2
  Constant1/1 -> Divide/2
  Multiply/1 -> Subsystem/1(In1), Integrator/1
  Linear n-th order actuator (SISO)1/1 -> Derivative2/1, Vector Concatenate1/1
  Linear n-th order actuator (SISO)2/1 -> Vector Concatenate2/1, Derivative/1
  position/1 -> Linear n-th order actuator (SISO)1/1
  Vector Concatenate1/1 -> Add2/1
  Vector Concatenate2/1 -> Add2/2
  Add2/1 -> Saturation/1
  Derivative2/1 -> Vector Concatenate1/2, Derivative3/1
  Derivative3/1 -> Vector Concatenate1/3
  Saturation/1 -> Gain12/1
  Subsystem/1(Out1) -> roll_angle/1
  Measure/1 -> Linear n-th order actuator (SISO)2/1

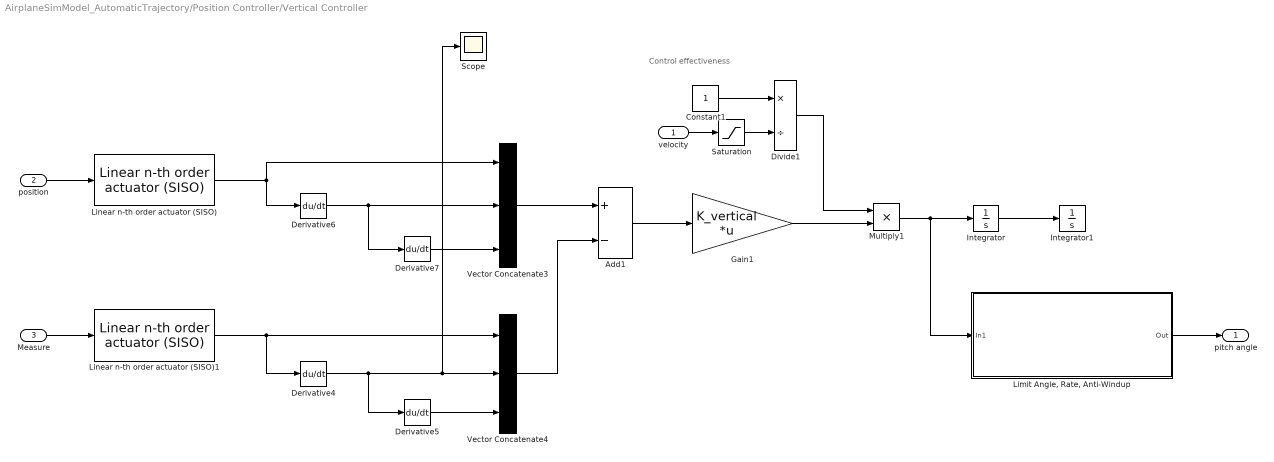
== system AirplaneSimModel_AutomaticTrajectory/Position Controller/Vertical Controller ==
  note: Control effectiveness
  velocity : Inport  PortDimensions=1
  position : Inport  Port=2  PortDimensions=1
  Measure : Inport  Port=3
  Add1 : Sum  Inputs=+-
  Constant1 : Constant
  Derivative{4..7} (4 alike) : Derivative
  Divide1 : Product  Inputs=*/
  Gain1 : Gain  Gain=K_vertical  Multiplication=Matrix(K*u)
  Integrator : Integrator
  Integrator1 : Integrator
  "Limit Angle, Rate, Anti-Windup" : Subsystem
  Linear n-th order actuator (SISO) : actuators_lib/Linear n-th order actuator (SISO)  omega=80  order=2  output_order=1  use_inital_value=on
      settings: SourceProductName=LADAC
  Linear n-th order actuator (SISO)1 : actuators_lib/Linear n-th order actuator (SISO)  omega=80  order=2  output_order=1  use_inital_value=on
      settings: SourceProductName=LADAC
  Multiply1 : Product
  Saturation : Saturate  UpperLimit=30  LowerLimit=5
  Scope : Scope
  Vector Concatenate3 : Concatenate  NumInputs=3
  Vector Concatenate4 : Concatenate  NumInputs=3
  pitch angle : Outport  PortDimensions=1
  wires:
  Linear n-th order actuator (SISO)1/1 -> Vector Concatenate4/1, Derivative4/1
  Gain1/1 -> Multiply1/2
  Derivative4/1 -> Derivative5/1, Scope/1, Vector Concatenate4/2
  Multiply1/1 -> "Limit Angle, Rate, Anti-Windup"/1(In1), Integrator/1
  Derivative5/1 -> Vector Concatenate4/3
  velocity/1 -> Saturation/1
  Constant1/1 -> Divide1/1
  Divide1/1 -> Multiply1/1
  Integrator/1 -> Integrator1/1
  Vector Concatenate3/1 -> Add1/1
  Vector Concatenate4/1 -> Add1/2
  Add1/1 -> Gain1/1
  Derivative6/1 -> Vector Concatenate3/2, Derivative7/1
  Measure/1 -> Linear n-th order actuator (SISO)1/1
  position/1 -> Linear n-th order actuator (SISO)/1
  Derivative7/1 -> Vector Concatenate3/3
  Linear n-th order actuator (SISO)/1 -> Vector Concatenate3/1, Derivative6/1
  "Limit Angle, Rate, Anti-Windup"/1(Out) -> pitch angle/1
  Saturation/1 -> Divide1/2

== system AirplaneSimModel_AutomaticTrajectory/QuaternionAttitudeController/DCM 2 q_bg continuous1 ==
  DCM : Inport
  DCM to quaternions : MATLAB Function  TreatAsAtomicUnit=on
  Delay : Delay  DelayLength=1  InitialConditionSource=Input port
      settings: InputPortMap=u0,p4
  MATLAB Function3 : MATLAB Function  TreatAsAtomicUnit=on
  quat : Outport
  wires:
  DCM to quaternions/1(q_bg) -> Delay/2
  MATLAB Function3/1(q_bg) -> quat/1, Delay/1  "q_bg"
  DCM/1 -> MATLAB Function3/1(M_bg), DCM to quaternions/1(M_bg)
  Delay/1 -> MATLAB Function3/2(last_q)

== system AirplaneSimModel_AutomaticTrajectory/QuaternionAttitudeController/DCM 2 q_bg continuous3 ==
  DCM : Inport
  DCM to quaternions : MATLAB Function  TreatAsAtomicUnit=on
  Delay : Delay  DelayLength=1  InitialConditionSource=Input port
      settings: InputPortMap=u0,p4
  MATLAB Function3 : MATLAB Function  TreatAsAtomicUnit=on
  quat : Outport
  wires:
  DCM to quaternions/1(q_bg) -> Delay/2
  MATLAB Function3/1(q_bg) -> quat/1, Delay/1  "q_bg"
  DCM/1 -> MATLAB Function3/1(M_bg), DCM to quaternions/1(M_bg)
  Delay/1 -> MATLAB Function3/2(last_q)

== system AirplaneSimModel_AutomaticTrajectory/QuaternionAttitudeController/DCM 2 q_bg continuous4 ==
  DCM : Inport
  DCM to quaternions : MATLAB Function  TreatAsAtomicUnit=on
  Delay : Delay  DelayLength=1  InitialConditionSource=Input port
      settings: InputPortMap=u0,p4
  MATLAB Function3 : MATLAB Function  TreatAsAtomicUnit=on
  quat : Outport
  wires:
  DCM to quaternions/1(q_bg) -> Delay/2
  MATLAB Function3/1(q_bg) -> quat/1, Delay/1  "q_bg"
  DCM/1 -> MATLAB Function3/1(M_bg), DCM to quaternions/1(M_bg)
  Delay/1 -> MATLAB Function3/2(last_q)

== system AirplaneSimModel_AutomaticTrajectory/QuaternionAttitudeController/Subsystem1 ==
  R : Inport
  alpha : Inport  Port=2
  roll angle : Inport  Port=3
  Constant16 : Constant  Value=0
  Euler Angles to Rotation Matrix : axes_transformation_lib/Euler Angles to Rotation Matrix  SystemSampleTime=-1
      settings: SourceProductName=LADAC
  Multiply2 : Product  Multiplication=Matrix(*)
  Vector Concatenate2 : Concatenate  NumInputs=3
  R_alpha : Outport
  wires:
  Multiply2/1 -> R_alpha/1
  Euler Angles to Rotation Matrix/1 -> Multiply2/2
  Vector Concatenate2/1 -> Euler Angles to Rotation Matrix/1
  R/1 -> Multiply2/1
  alpha/1 -> Vector Concatenate2/2
  Constant16/1 -> Vector Concatenate2/3
  roll angle/1 -> Vector Concatenate2/1

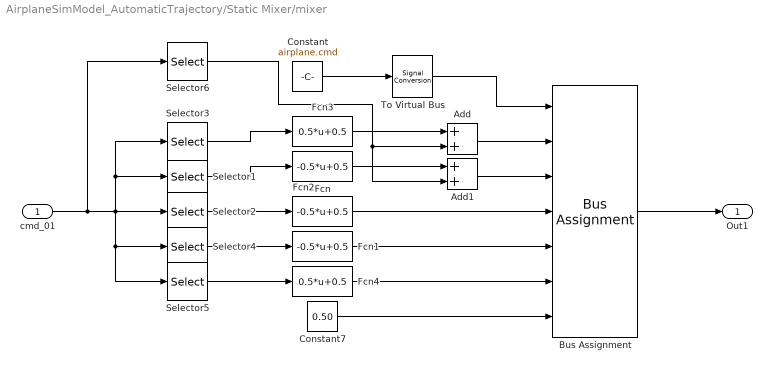
== system AirplaneSimModel_AutomaticTrajectory/Static Mixer/mixer ==
  cmd_01 : Inport
  Add : Sum
  Add1 : Sum
  Bus Assignment : BusAssignment  AssignedSignals=aileron_left,aileron_right,elevator,rudder,throttle,htp_trim
  Constant : Constant  Value=airplane.cmd  OutDataTypeStr=Bus: cmdBus
  Constant7 : Constant  Value=0.50
  Fcn : Fcn  Expr=-0.5*u+0.5
  Fcn1 : Fcn  Expr=-0.5*u+0.5
  Fcn2 : Fcn  Expr=-0.5*u+0.5
  Fcn3 : Fcn  Expr=0.5*u+0.5
  Fcn4 : Fcn  Expr=0.5*u+0.5
  Selector1 : Selector  InputPortWidth=8  IndexOptions=Index vector (dialog)  Indices=1  OutputSizes=1
  Selector2 : Selector  InputPortWidth=8  IndexOptions=Index vector (dialog)  Indices=2  OutputSizes=1
  Selector3 : Selector  InputPortWidth=8  IndexOptions=Index vector (dialog)  Indices=1  OutputSizes=1
  Selector4 : Selector  InputPortWidth=8  IndexOptions=Index vector (dialog)  Indices=3  OutputSizes=1
  Selector5 : Selector  InputPortWidth=8  IndexOptions=Index vector (dialog)  Indices=4  OutputSizes=1
  Selector6 : Selector  InputPortWidth=8  IndexOptions=Index vector (dialog)  Indices=5  OutputSizes=1
  To Virtual Bus : SignalConversion  ConversionOutput=Virtual bus  OverrideOpt=off
  Out1 : Outport
  wires:
  Constant/1 -> To Virtual Bus/1
  Bus Assignment/1 -> Out1/1
  cmd_01/1 -> Selector6/1, Selector2/1, Selector5/1, Selector4/1, Selector1/1, Selector3/1
  Selector4/1 -> Fcn1/1
  Selector2/1 -> Fcn2/1
  Selector1/1 -> Fcn/1
  Selector3/1 -> Fcn3/1
  Selector5/1 -> Fcn4/1
  Constant7/1 -> Bus Assignment/7
  Fcn1/1 -> Bus Assignment/5
  To Virtual Bus/1 -> Bus Assignment/1
  Fcn2/1 -> Bus Assignment/4
  Fcn4/1 -> Bus Assignment/6
  Add/1 -> Bus Assignment/2
  Add1/1 -> Bus Assignment/3
  Fcn3/1 -> Add/1
  Fcn/1 -> Add1/1
  Selector6/1 -> Add1/2, Add/2

== system AirplaneSimModel_AutomaticTrajectory/scopes/actuator scopes ==
  actuatorBus : Inport
  Bus Selector : BusSelector  OutputSignals=aileronsBus.deflection_in_rad,elevatorBus.deflection_in_rad,rudderBus.deflection_in_rad,htpTrimBus.deflection_in_rad,motorBus.angular_velocity_in_rad_per_s
  ailerons : Scope
  elevator : Scope
  htpTrim : Scope
  motor : Scope
  rudder : Scope
  wires:
  actuatorBus/1 -> Bus Selector/1
  Bus Selector/1 -> ailerons/1  "<deflection_in_rad>"
  Bus Selector/2 -> elevator/1  "<deflection_in_rad>"
  Bus Selector/3 -> rudder/1  "<deflection_in_rad>"
  Bus Selector/4 -> htpTrim/1  "<deflection_in_rad>"
  Bus Selector/5 -> motor/1  "<angular_velocity_in_rad_per_s>"

== system AirplaneSimModel_AutomaticTrajectory/scopes/aero scopes ==
  aeroBus : Inport
  Bus Selector : BusSelector  OutputSignals=aeroMainWing,aeroHtp,aerVtp,aeroFuse
  Bus Selector1 : BusSelector  OutputSignals=R_Ab,Q_Ab
  Scope : Scope
  Scope1 : Scope
  Subsystem : Subsystem
  Subsystem1 : Subsystem
  Subsystem2 : Subsystem
  wires:
  aeroBus/1 -> Bus Selector/1
  Bus Selector/1 -> Subsystem/1(In1)  "<aeroMainWing>"
  Bus Selector/2 -> Subsystem1/1(In1)  "<aeroHtp>"
  Bus Selector/3 -> Subsystem2/1(In1)  "<aerVtp>"
  Bus Selector/4 -> Bus Selector1/1  "<aeroFuse>"
  Bus Selector1/1 -> Scope/1  "<R_Ab>"
  Bus Selector1/2 -> Scope1/1  "<Q_Ab>"

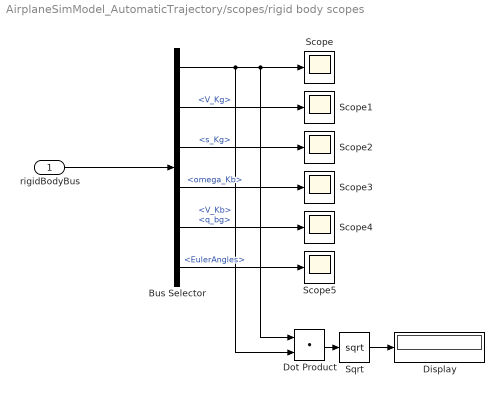
== system AirplaneSimModel_AutomaticTrajectory/scopes/rigid body scopes ==
  rigidBodyBus : Inport
  Bus Selector : BusSelector  OutputSignals=V_Kb,V_Kg,s_Kg,omega_Kb,q_bg,EulerAngles
  Display : Display
  Dot Product : DotProduct  InputSameDT=on  OutDataTypeStr=Inherit: Inherit via internal rule
  Scope{,1..5} (6 alike) : Scope
  Sqrt : Sqrt  SaturateOnIntegerOverflow=on
  wires:
  rigidBodyBus/1 -> Bus Selector/1
  Bus Selector/1 -> Dot Product/2, Dot Product/1, Scope/1  "<V_Kb>"
  Bus Selector/2 -> Scope1/1  "<V_Kg>"
  Bus Selector/3 -> Scope2/1  "<s_Kg>"
  Bus Selector/4 -> Scope3/1  "<omega_Kb>"
  Bus Selector/5 -> Scope4/1  "<q_bg>"
  Bus Selector/6 -> Scope5/1  "<EulerAngles>"
  Dot Product/1 -> Sqrt/1
  Sqrt/1 -> Display/1

== system AirplaneSimModel_AutomaticTrajectory/Position Controller/Lateral Controller/Subsystem ==
  In1 : Inport
  Integrator1 : Integrator  LimitOutput=on  UpperSaturationLimit=45/57.3  LowerSaturationLimit=-45/57.3
  Saturation : Saturate  UpperLimit=5  LowerLimit=-5
  Scope : Scope  NumInputPorts=2
  Out1 : Outport
  wires:
  In1/1 -> Saturation/1
  Saturation/1 -> Integrator1/1, Scope/1
  Integrator1/1 -> Out1/1, Scope/2

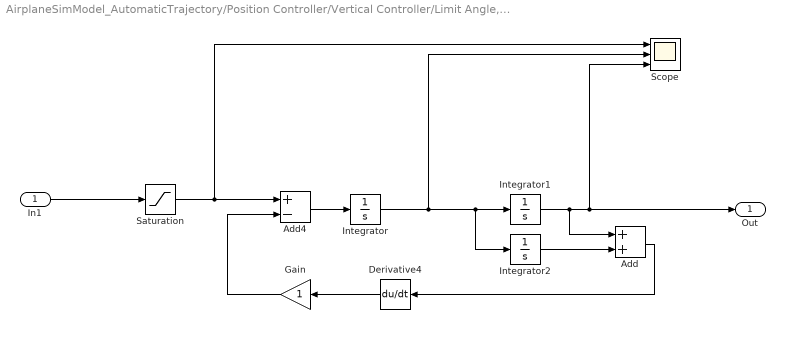
== system AirplaneSimModel_AutomaticTrajectory/Position Controller/Vertical Controller/Limit Angle, Rate, Anti-Windup ==
  In1 : Inport
  Add : Sum
  Add4 : Sum  Inputs=+-
  Derivative4 : Derivative
  Gain : Gain
  Integrator : Integrator  LimitOutput=on  UpperSaturationLimit=0.8  LowerSaturationLimit=-0.8
  Integrator1 : Integrator  LimitOutput=on  UpperSaturationLimit=45/57.3  LowerSaturationLimit=-45/57.3
  Integrator2 : Integrator
  Saturation : Saturate  UpperLimit=5  LowerLimit=-5
  Scope : Scope  NumInputPorts=3
  Out : Outport
  wires:
  Gain/1 -> Add4/2
  Integrator1/1 -> Scope/3, Out/1, Add/1
  Derivative4/1 -> Gain/1
  Add/1 -> Derivative4/1
  In1/1 -> Saturation/1
  Add4/1 -> Integrator/1
  Integrator2/1 -> Add/2
  Integrator/1 -> Scope/2, Integrator2/1, Integrator1/1
  Saturation/1 -> Scope/1, Add4/1

== system AirplaneSimModel_AutomaticTrajectory/scopes/aero scopes/Subsystem ==
  In1 : Inport
  Bus Selector : BusSelector  OutputSignals=aeroAxes.alpha_M_P,aeroAxes.beta_M_P,aeroAxes.q_P,dynamicsBody.R_Ab,dynamicsBody.Q_Ab,dynamicsBody.xyz_np_b,dynamicsBody.C_m_camber_np_b
  Scope{,1..6} (7 alike) : Scope
  rad2deg : unit_conversions_lib/rad2deg
      settings: SourceProductName=LADAC
  wires:
  In1/1 -> Bus Selector/1
  Bus Selector/1 -> rad2deg/1  "<alpha_M_P>"
  Bus Selector/3 -> Scope2/1  "<q_P>"
  Bus Selector/2 -> Scope1/1  "<beta_M_P>"
  Bus Selector/4 -> Scope3/1  "<R_Ab>"
  Bus Selector/5 -> Scope4/1  "<Q_Ab>"
  Bus Selector/6 -> Scope5/1  "<xyz_np_b>"
  Bus Selector/7 -> Scope6/1  "<C_m_camber_np_b>"
  rad2deg/1 -> Scope/1

== system AirplaneSimModel_AutomaticTrajectory/scopes/aero scopes/Subsystem1 ==
  In1 : Inport
  Bus Selector : BusSelector  OutputSignals=aeroAxes.alpha_M_P,aeroAxes.beta_M_P,aeroAxes.q_P,dynamicsBody.R_Ab,dynamicsBody.Q_Ab
  Scope{,1..4} (5 alike) : Scope
  rad2deg : unit_conversions_lib/rad2deg
      settings: SourceProductName=LADAC
  wires:
  Bus Selector/5 -> Scope4/1  "<Q_Ab>"
  Bus Selector/4 -> Scope3/1  "<R_Ab>"
  Bus Selector/2 -> Scope1/1  "<beta_M_P>"
  Bus Selector/3 -> Scope2/1  "<q_P>"
  Bus Selector/1 -> rad2deg/1  "<alpha_M_P>"
  In1/1 -> Bus Selector/1
  rad2deg/1 -> Scope/1

== system AirplaneSimModel_AutomaticTrajectory/scopes/aero scopes/Subsystem2 ==
  In1 : Inport
  Bus Selector : BusSelector  OutputSignals=aeroAxes.alpha_M_P,aeroAxes.beta_M_P,aeroAxes.q_P,dynamicsBody.R_Ab,dynamicsBody.Q_Ab
  Scope{,1..4} (5 alike) : Scope
  wires:
  In1/1 -> Bus Selector/1
  Bus Selector/1 -> Scope/1  "<alpha_M_P>"
  Bus Selector/3 -> Scope2/1  "<q_P>"
  Bus Selector/2 -> Scope1/1  "<beta_M_P>"
  Bus Selector/4 -> Scope3/1  "<R_Ab>"
  Bus Selector/5 -> Scope4/1  "<Q_Ab>"

== matlab function AirplaneSimModel_AutomaticTrajectory/QuaternionAttitudeController/DCM 2 q_bg continuous4/DCM to quaternions ==
  data: M_bg input; q_bg output
function q_bg  = fcn( M_bg ) %#codegen
q_bg  = rotm2quat( M_bg );

== matlab function AirplaneSimModel_AutomaticTrajectory/MatchAircraftToTrajectory/MATLAB Function6 ==
  data: pos output; error output; error_vec output; traj input; pos_ac input; section_idx output; t output; vel input; vel_dt input; acc_vec input; use_iterative_algo input; acc output; M_tg output; dt output; pos_dt output; pos_dt2 output
function [pos, error, error_vec, section_idx, t, acc, M_tg, dt, pos_dt, pos_dt2]  = GetMatch(traj, pos_ac, vel, vel_dt, acc_vec, use_iterative_algo)

section_idx = 1;
t = 0;

if use_iterative_algo 
     [section_idx, ~, t] = trajGetMatchEnhanced(traj, pos_ac, section_idx);
else
     [section_idx, ~, t] = trajGetMatch(traj, pos_ac, section_idx);
end

traj_section = trajGetSection(traj, section_idx);

pos = trajSectionGetPos(traj_section, t);

error_vec = (pos - pos_ac);

error = norm(error_vec);

[T, B, N, kappa, tau] = trajSectionGetFrenetSerretWithAcceleration(traj_section, vel, acc_vec, t);

% Calculate path acceleration
acc = (kappa * N) * vel^2;

M_tg = [T, B, -N];

%%

[first_deriv, sec_deriv, ~] = trajSectionGetDerivatives(traj_section, t);

% Derivative of arc length in respect to dt
ds_dt = norm(first_deriv);
ds_dt2 = norm(sec_deriv);

% Rate of change of t
dt =  vel / max(ds_dt, eps);
dt2 =  vel_dt / max(ds_dt, eps);

pos_dt  = first_deriv * dt;
pos_dt2 = sec_deriv * dt + first_deriv * dt2;


%[T, B, N, kappa, tau] = trajSectionGetFrenetSerretWithAcceleration(active_section, vel, [0; 0; 0], t);

%Darboux vector
% daboux_vec = tau*T + kappa*B;
% 
% dot_T = cross(daboux_vec, T);
% dot_B = cross(daboux_vec, B);
% dot_N = cross(daboux_vec, N);
% 
% dot_M_tg = [dot_T, dot_B, dot_N];
% 
% omega = [dot_M_tg(1, 2); dot_M_tg(1, 3); kappa - (9.81/vel^2)];


end

== matlab function AirplaneSimModel_AutomaticTrajectory/QuaternionAttitudeController/DCM 2 q_bg continuous1/DCM to quaternions ==
  data: M_bg input; q_bg output
function q_bg  = fcn( M_bg ) %#codegen
q_bg  = rotm2quat( M_bg );

== matlab function AirplaneSimModel_AutomaticTrajectory/QuaternionAttitudeController/DCM 2 q_bg continuous1/MATLAB Function3 ==
  data: M_bg input; q_bg output; last_q input
function q_bg  = dcm2QuatCont( M_bg, last_q )

% dcm2Quat computes the quaternion (q_bg) from the direction cosine matrix
% (DCM) so that there are no discontinuities.
%   The quaternion is used to represent the attitude of the body
%   relative to the earth. It can be computed from the DCM. However, there
%   exist two solutions with reversed signs. This function avoids steps
%   which can be important for controllers.
% 
% Literature:
%   [1] Wu, J. (2018). Optimal Continuous Unit Quaternions from Rotation
%       Matrices. Journal of Guidance, Control and Dynamics.
% 
% Inputs:
%   M_bg            direction cosine matrix (with 3x3 elements) from NED
%                   frame (g) to body frame (b).
% 
% Outputs:
%   q_bg            quaternion vector with 4 elements and euclean norm of 1
% 
% See also: dcm2Quat
% 

% Disclamer:
%   SPDX-License-Identifier: GPL-2.0-only
% 
%   Copyright (C) 2020-2022 Yannic Beyer
%   Copyright (C) 2022 TU Braunschweig, Institute of Flight Guidance
% *************************************************************************

% get quaternions (with discontinuities)

%q_bg = dcm2Quat( M_bg );
q_bg = rotm2quat(M_bg)';

% remove discontinuities
q_bg = sign(q_bg' * last_q) * q_bg;


end

== matlab function AirplaneSimModel_AutomaticTrajectory/QuaternionAttitudeController/DCM 2 q_bg continuous3/DCM to quaternions ==
  data: M_bg input; q_bg output
function q_bg  = fcn( M_bg ) %#codegen
q_bg  = rotm2quat( M_bg );

== matlab function AirplaneSimModel_AutomaticTrajectory/QuaternionAttitudeController/DCM 2 q_bg continuous3/MATLAB Function3 ==
  data: M_bg input; q_bg output; last_q input
function q_bg  = dcm2QuatCont( M_bg, last_q )

% dcm2Quat computes the quaternion (q_bg) from the direction cosine matrix
% (DCM) so that there are no discontinuities.
%   The quaternion is used to represent the attitude of the body
%   relative to the earth. It can be computed from the DCM. However, there
%   exist two solutions with reversed signs. This function avoids steps
%   which can be important for controllers.
% 
% Literature:
%   [1] Wu, J. (2018). Optimal Continuous Unit Quaternions from Rotation
%       Matrices. Journal of Guidance, Control and Dynamics.
% 
% Inputs:
%   M_bg            direction cosine matrix (with 3x3 elements) from NED
%                   frame (g) to body frame (b).
% 
% Outputs:
%   q_bg            quaternion vector with 4 elements and euclean norm of 1
% 
% See also: dcm2Quat
% 

% Disclamer:
%   SPDX-License-Identifier: GPL-2.0-only
% 
%   Copyright (C) 2020-2022 Yannic Beyer
%   Copyright (C) 2022 TU Braunschweig, Institute of Flight Guidance
% *************************************************************************

% get quaternions (with discontinuities)

%q_bg = dcm2Quat( M_bg );
q_bg = rotm2quat(M_bg)';

% remove discontinuities
q_bg = sign(q_bg' * last_q) * q_bg;


end
